simulink model "model_line_detector_2"  (R2023a)
settings: Solver=VariableStepAuto  StartTime=0.0  StopTime=25  RelTol=1e-3
model workspace (MAT data in the model file):
  BusActorsActors = canlib.Parameter
  BusActorsActors.DataType = 'auto'
  BusActorsActors.Complexity = 'real'
  BusActorsActors.Dimensions = [0 0]
values from neighbouring files (symbols this model uses):
  A = [a11 a12 ... (first row only)    [model.m]
  af = 1.104    [calc_Kvar.m]    (also in model.m)
  B = [b11 b12 ... (first row only)    [model.m]
  C = [1 0 ... (first row only)    [calc_Kvar.m]    (also in model.m)
  D = [0 0;0 0]    [calc_Kvar.m]    (also in model.m)
  E = [e1 ... (first row only)    [model.m]
  x0 = [0; 0]    [model.m]
undefined symbols (not defined in the file or in its folder): calc_A, calc_B, calc_E, calc_fb, calc_ff, driving, sigbuilder_block
libraries: drivingscenarioandsensors x2
settings Model: PacingRate=2  Creator=Utente  LastModifiedBy=Ferna
settings SolverCC: AlgebraicLoopSolver=TrustRegion
settings DebuggingCC: UnconnectedInputMsg=warning  UnconnectedOutputMsg=warning  UnconnectedLineMsg=warning
settings ModelReferenceCC: EnableRefExpFcnMdlSchedulingChecks=on
settings RTWCC: DLArmComputeVersion=19.05

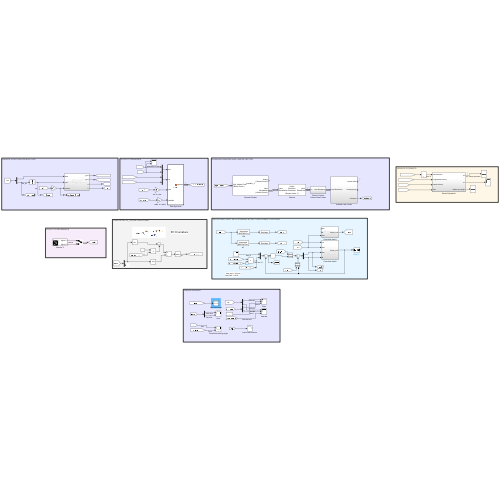
[thumbnail: Simulink's stored preview of the top-level diagram]
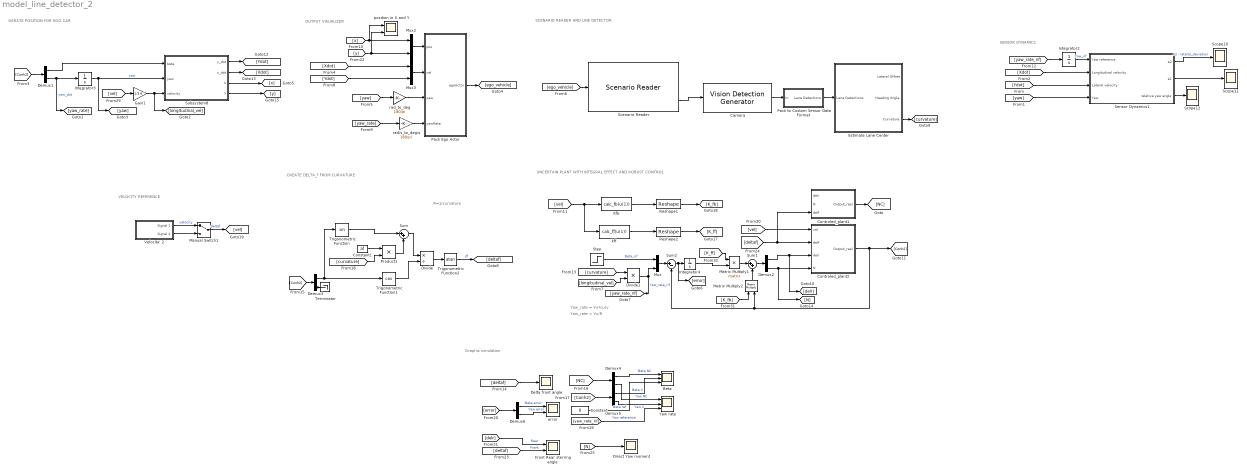
== system model_line_detector_2 ==
  note: Graphis simulation
  note: VELOCITY REFERENCE
  note: GERATE POSITION FOR EGO CAR
  note: UNCERTAIN PLANT WITH INTEGRAL EFFECT AND ROBUST CONTROL
  note: CREATE DELTA_f FROM CURVATURE
  note: SCENARIO READER AND LINE DETECTOR
  note: Yaw_rate = Vx*curv
  note: Yaw_rate = Vx/R
  note: SENSOR DYNAMICS
  note: OUTPUT VISUALIZER
  note: R=1/curvature
  Beta : Scope  NumInputPorts=3
  Camera : drivingscenarioandsensors/Vision Detection Generator  SensorIndex=1  DetectorOutput=Lanes only  UpdateInterval=0.01  LaneUpdateInterval=0.1  SensorLocation=[1.9 0]  Height=1.1  Yaw=0  Pitch=1  Roll=0  BusNameSource=Auto  BusName=BusObjectDetections  BusName2Source=Property  BusName2=BusVision  MaxNumDetectionsSource=Property  MaxNumDetections=50  MaxNumLanesSource=Property  MaxNumLanes=2  DetectionCoordinates=Ego Cartesian  SimulateUsing=Interpreted execution  MaxRange=50  BoundingBoxAccuracy=5  ProcessNoiseIntensity=5  MaxSpeed=50  MaxAllowedOcclusion=0.5  MinObjectImageSize=[15 15]  DetectionProbability=0.9  FalsePositivesPerImage=0.1  MinLaneImageSize=[20 3]  LaneBoundaryAccuracy=3  HasNoise=on  InitialSeedSource=Specify seed  InitialSeed=0  UsedSeed=0  ActorProfilesSource=Parameters  ActorProfilesParameters=driving.internal.ActorProfilesParameters  ActorProfilesExpression=[struct('ActorID',1,'ClassID',1,'Length',4.7,'Width',1.8,'Height',1.4,'OriginOffset',[-1.35 0 0],'MeshVertices',[3.7 -0.9 1.4;3.7 0.9 1.4;-1 0.9 1.4;-1 -0.9 1.4;3.7 -0.9 0;3.7 0.9 0;-1 0.9 0;-1 -0.9 0],'MeshFaces',[6 2 1;1 5 6;8 4 3;3 7 8;6 7 3;3 2 6;5 1 4;4 8 5;4 1 2;2 3 4;7 6 5;5 8 7],'RCSPattern',[10 10;10 10],'RCSAzimuthAngles',[-180 180],'RCSElevationAngles',[-90 90])]  Intrinsics=driving.internal.cameraIntrinsics('FocalLength',[800 799.999999999999],'PrincipalPoint',[320 240],'ImageSize',[480 640],'RadialDistortion',[0 0],'TangentialDistortion',[0 0],'Skew',0)
  Constant : Constant  Value=0
  Constant1 : Constant  Value=af
  Controled_plant1 : Subsystem
  Controled_plant2 : Subsystem
  Delta front angle : Scope
  Demux{1..6} (6 alike) : Demux  Outputs=2
  Direct Yaw moment : Scope
  Divide : Product  Inputs=*/
  Divide1 : Product  Inputs=**
  Estimate Lane Center : Subsystem  VariantControl=v2
  Front Rear sterring angle : Scope  NumInputPorts=2
  Gain1 : Gain  Gain=1/3.6
  Integrator2 : Integrator
  Integrator3 : Integrator  InitialCondition=0 %0.5411
  Integrator4 : Integrator
  Kfb : MATLABFcn  MATLABFcn=calc_fb(u(1))
  Manual Switch1 : ManualSwitch
  Matrix Multiply1 : Product  Multiplication=Matrix(*)
  Matrix Multiply2 : Product  Multiplication=Matrix(*)
  Mux : Mux  Inputs=2
  Mux2 : Mux  Inputs=2
  Mux3 : Mux  Inputs=2
  Pack Ego Actor : MATLAB Function  TreatAsAtomicUnit=on
  Pack to Custom Sensor Data Format : Subsystem
  Product1 : Product
  Reshape1 : Reshape  OutputDimensionality=Customize  OutputDimensions=[2,2]
  Reshape2 : Reshape  OutputDimensionality=Customize  OutputDimensions=[2,2]
  Scenario Reader : drivingscenarioandsensors/Scenario Reader  ScenarioSource=From file  ScenarioFileName=C:\Users\Ferna\Desktop\MASTER\third semester\vehicle control\proyectos\Vehicle control Mod_2 MIO\matlab\scenario_2.mat  ScenarioVariableName=scenario  OutputCoordinateSystem=Vehicle coordinates  EgoVehicleSource=Input port  EgoVehicleActorID=1  OrientVehiclesOnRoad=off  OutputEgoVehiclePose=off  OutputEgoVehicleState=off  SampleTime=0.1  LaneBoundaryOutput=Ego vehicle lane boundaries  LaneBoundaryDistance=linspace(-150, 150, 1500)  LaneBoundaryLocation=Center of lane markings  BusNameSource=Auto  BusName=BusActors  BusNumActorsSource=Scenario  BusNumActors=100  BusName2Source=Auto  BusName2=BusLaneBoundaries  BusNumLaneBoundariesSource=Scenario  BusNumLaneBoundaries=10  BusName3Source=Auto  BusName3=BusEgoActor  BusName4Source=Auto  BusName4=BusEgoState  ShowCoordinateLabels=on  SimulateUsing=Interpreted execution
  Scope10 : Scope
  Scope11 : Scope
  Scope12 : Scope
  Sensor Dynamics1 : Subsystem
  Step : Step  After=0  SampleTime=0
  Subsystem8 : Subsystem
  Sum : Sum  Inputs=|++
  Sum1 : Sum  Inputs=|++
  Sum2 : Sum  Inputs=|+-
  Terminator : Terminator
  Trigonometric Function : Trigonometry
  Trigonometric Function1 : Trigonometry  Operator=cos
  Trigonometric Function2 : Trigonometry  Operator=atan
  Velocita' 2 : Subsystem  Tag=STV Subsys  LoadFcn=sigbuilder_block('load');  StartFcn=sigbuilder_block('start');  StopFcn=sigbuilder_block('stop');  ClipboardFcn=sigbuilder_block('clipboard');  mask(Sigbuilder block){tuvar=[0:10]}
      mask help: Simulink:masks:SigbuilderBlock_MD
      mask init:
      | if ~strcmp(get_param(bdroot(gcbh),'SimulationStatus'),'stopped') tuvar = sigbuilder_block('maskInit'); end
      settings: CopyFcn=sigbuilder_block('copy');  DeleteFcn=sigbuilder_block('delete');  ModelCloseFcn=sigbuilder_block('modelClose');  PreSaveFcn=sigbuilder_block('preSave');  PauseFcn=sigbuilder_block('pause');  ContinueFcn=sigbuilder_block('continue');  NameChangeFcn=sigbuilder_block('namechange');  OpenFcn=sigbuilder_block('open',[5.4 36 1141.2 516.6 ]);  CloseFcn=sigbuilder_block('close');
      mask Display: plot(0, 0, 100, 100,[2, 2, 32, 32, 2], [68, 8, 8, 68, 68],[32, 2], [38, 38], [32, 19, 2],[53, 60, 44], [32, 17, 17, 2],[16, 16, 31, 31]);txt = getActiveGroup(gcbh);text(2, 100, txt,'verticalAlignment', 'top');
  Yaw rate : Scope  NumInputPorts=3
  error : Scope  NumInputPorts=2
  kff : MATLABFcn  MATLABFcn=calc_ff(u(1))
  position in X and Y : Scope  NumInputPorts=2
  rad/s_to_deg/s : Gain  Gain=180/pi
  "rad_to_deg  " : Gain  Gain=180/pi
  wires:
  [Xdot] -> Sensor Dynamics1/2(Longitudinal velocity)
  [Ydot] -> Sensor Dynamics1/3(Lateral velocity)
  [yaw] -> Sensor Dynamics1/4("Yaw ")
  Mux2/1 -> Pack Ego Actor/1(pos)
  [Xdot] -> Mux3/1
  Mux3/1 -> Pack Ego Actor/2(vel)
  [yaw] -> "rad_to_deg  "/1
  Pack Ego Actor/1(egoActor) -> [ego_vehicle]
  [yaw_rate] -> rad/s_to_deg/s/1
  "rad_to_deg  "/1 -> Pack Ego Actor/3(yaw)
  [Ydot] -> Mux3/2
  rad/s_to_deg/s/1 -> Pack Ego Actor/4(yawRate)
  [x] -> position in X and Y/1, Mux2/1
  [y] -> Mux2/2, position in X and Y/2
  Camera/1 -> Pack to Custom Sensor Data Format/1(In)
  Scenario Reader/2 -> Camera/1
  Pack to Custom Sensor Data Format/1(Lane Detections) -> Estimate Lane Center/1(Lane Detections)
  [ego_vehicle] -> Scenario Reader/1
  Divide1/1 -> [yaw_rate_rif], Mux/2  "Yaw_rate_rif"
  Estimate Lane Center/3(" Curvature") -> [curvature]
  Integrator2/1 -> Sensor Dynamics1/1(Yaw reference)  "Yaw_rif"
  [longitudinal_vel] -> Divide1/2
  Sensor Dynamics1/1(e2) -> Scope10/1  "e2 - lateral_deviation"
  Subsystem8/1(y_dot) -> [Ydot]
  Gain1/1 -> [longitudinal_vel], Subsystem8/3(velocity)
  Sensor Dynamics1/2(e1) -> Scope11/1
  Sensor Dynamics1/3(relative yaw angle) -> Scope12/1
  Demux2/2 -> [N], Controled_plant2/4(N)
  [deltaf] -> Controled_plant1/3(delf), Controled_plant2/2(delf)
  Matrix Multiply1/1 -> Sum1/1
  Demux2/1 -> [delr], Controled_plant2/3(delr)
  Sum2/1 -> [error], Integrator4/1
  Sum1/1 -> Demux2/1
  Controled_plant2/1(Output_real) -> Sum2/2, Matrix Multiply2/2, [Conh2]
  Controled_plant1/1(Output_real) -> [NC]
  Integrator4/1 -> Matrix Multiply1/2
  Demux3/2 -> Terminator/1
  Demux1/1 -> Subsystem8/1(beta)
  Demux1/2 -> [yaw_rate], Integrator3/1  "yaw_dot"
  Integrator3/1 -> [yaw], Subsystem8/2(yaw)  "yaw"
  Subsystem8/2(x_dot) -> [Xdot]
  Subsystem8/3(X) -> [x]
  Subsystem8/4(Y) -> [y]
  Mux/1 -> Sum2/1
  Step/1 -> Mux/1  "Beta_rif"
  [Conh2] -> Demux1/1
  [Conh2] -> Demux3/1
  Reshape2/1 -> [K_ff]
  [vel] -> Gain1/1
  [K_fb] -> Matrix Multiply2/1
  Matrix Multiply2/1 -> Sum1/2
  [vel] -> Controled_plant2/1(vel)
  Reshape1/1 -> [K_fb]
  [K_ff] -> Matrix Multiply1/1
  [vel] -> kff/1, Kfb/1
  Kfb/1 -> Reshape1/1
  kff/1 -> Reshape2/1
  Velocita' 2/1(Signal 1) -> Manual Switch1/1  "velocity"
  Velocita' 2/2(Signal 2) -> Manual Switch1/2
  Manual Switch1/1 -> [vel]  "deltaf"
  [curvature] -> Divide1/1
  Trigonometric Function1/1 -> Divide/2
  Product1/1 -> Sum/2
  Constant1/1 -> Product1/1
  Trigonometric Function/1 -> Sum/1
  [curvature] -> Product1/2
  Trigonometric Function2/1 -> [deltaf]  "df"
  Demux3/1 -> Trigonometric Function/1, Trigonometric Function1/1
  Sum/1 -> Divide/1
  Divide/1 -> Trigonometric Function2/1
  [yaw_rate_rif] -> Integrator2/1
  [deltaf] -> Delta front angle/1
  [NC] -> Demux4/1
  [Conh2] -> Demux5/1
  Demux4/1 -> Beta/1  "Beta NC"
  Demux5/1 -> Beta/2  "Beta C"
  Constant/1 -> Beta/3  "Beta ref"
  Demux4/2 -> Yaw rate/1  "Yaw NC"
  Demux5/2 -> Yaw rate/2  "Yaw C"
  [yaw_rate_rif] -> Yaw rate/3  "Yaw reference"
  [error] -> Demux6/1
  Demux6/1 -> error/1  "Beta error"
  Demux6/2 -> error/2  "Yaw error"
  [delr] -> Front Rear sterring angle/1  "Rear"
  [deltaf] -> Front Rear sterring angle/2  "Front"
  [N] -> Direct Yaw moment/1

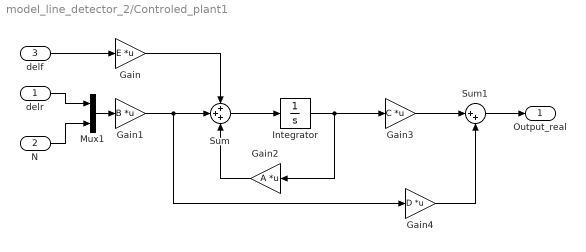
== system model_line_detector_2/Controled_plant1 ==
  delr : Inport
  N : Inport  Port=2
  delf : Inport  Port=3
  Gain : Gain  Gain=E  Multiplication=Matrix(K*u)
  Gain1 : Gain  Gain=B  Multiplication=Matrix(K*u)
  Gain2 : Gain  Gain=A  Multiplication=Matrix(K*u)
  Gain3 : Gain  Gain=C  Multiplication=Matrix(K*u)
  Gain4 : Gain  Gain=D  Multiplication=Matrix(K*u)
  Integrator : Integrator  InitialCondition=x0
  Mux1 : Mux  Inputs=2
  Sum : Sum  Inputs=+++
  Sum1 : Sum  Inputs=|++
  Output_real : Outport
  wires:
  Gain2/1 -> Sum/3
  Sum/1 -> Integrator/1
  Mux1/1 -> Gain1/1
  N/1 -> Mux1/2
  Gain3/1 -> Sum1/1
  Sum1/1 -> Output_real/1
  Gain/1 -> Sum/1
  Integrator/1 -> Gain2/1, Gain3/1
  delf/1 -> Gain/1
  delr/1 -> Mux1/1
  Gain4/1 -> Sum1/2
  Gain1/1 -> Sum/2, Gain4/1

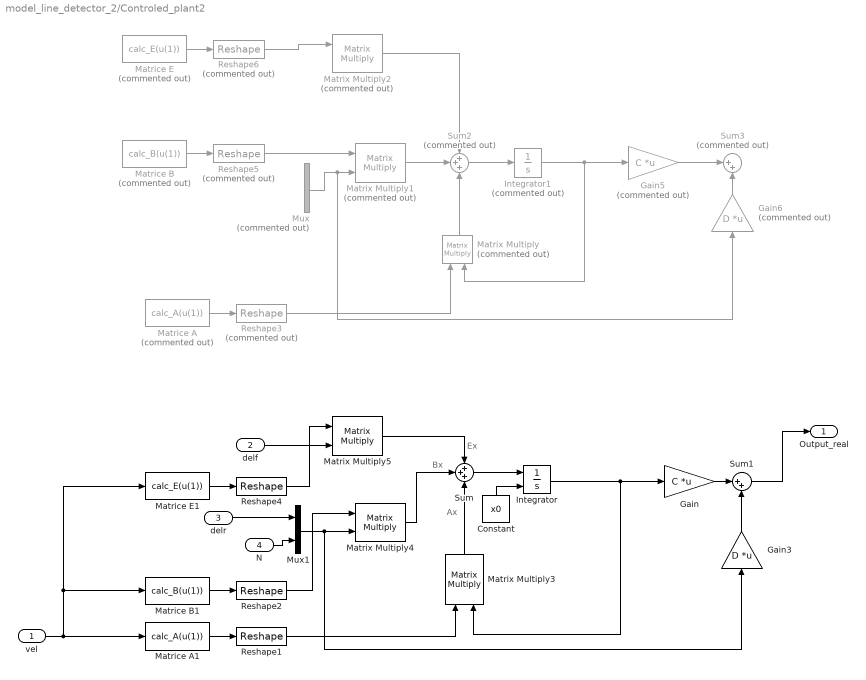
== system model_line_detector_2/Controled_plant2 ==
  note: Ex
  note: Bx
  note: Ax
  vel : Inport
  delf : Inport  Port=2
  delr : Inport  Port=3
  N : Inport  Port=4
  Constant : Constant  Value=x0
  Gain : Gain  Gain=C  Multiplication=Matrix(K*u)
  Gain3 : Gain  Gain=D  Multiplication=Matrix(K*u)
  Gain5 : Gain  Commented=on  Gain=C  Multiplication=Matrix(K*u)
  Gain6 : Gain  Commented=on  Gain=D  Multiplication=Matrix(K*u)
  Integrator : Integrator  InitialConditionSource=external
  Integrator1 : Integrator  Commented=on  InitialCondition=x0
  Matrice A : MATLABFcn  Commented=on  MATLABFcn=calc_A(u(1))
  Matrice A1 : MATLABFcn  MATLABFcn=calc_A(u(1))
  Matrice B : MATLABFcn  Commented=on  MATLABFcn=calc_B(u(1))
  Matrice B1 : MATLABFcn  MATLABFcn=calc_B(u(1))
  Matrice E : MATLABFcn  Commented=on  MATLABFcn=calc_E(u(1))
  Matrice E1 : MATLABFcn  MATLABFcn=calc_E(u(1))
  Matrix Multiply : Product  Commented=on  Multiplication=Matrix(*)
  Matrix Multiply1 : Product  Commented=on  Multiplication=Matrix(*)
  Matrix Multiply2 : Product  Commented=on  Multiplication=Matrix(*)
  Matrix Multiply3 : Product  Multiplication=Matrix(*)
  Matrix Multiply4 : Product  Multiplication=Matrix(*)
  Matrix Multiply5 : Product  Multiplication=Matrix(*)
  Mux : Mux  Commented=on  Inputs=2
  Mux1 : Mux  Inputs=2
  Reshape1 : Reshape  OutputDimensionality=Customize  OutputDimensions=[2,2]
  Reshape2 : Reshape  OutputDimensionality=Customize  OutputDimensions=[2,2]
  Reshape3 : Reshape  Commented=on  OutputDimensionality=Customize  OutputDimensions=[2,2]
  Reshape4 : Reshape  OutputDimensionality=Customize  OutputDimensions=[2,1]
  Reshape5 : Reshape  Commented=on  OutputDimensionality=Customize  OutputDimensions=[2,2]
  Reshape6 : Reshape  Commented=on  OutputDimensionality=Customize  OutputDimensions=[2,1]
  Sum : Sum  Inputs=+++
  Sum1 : Sum  Inputs=|++
  Sum2 : Sum  Commented=on  Inputs=+++
  Sum3 : Sum  Commented=on  Inputs=|++
  Output_real : Outport
  wires:
  Matrice E/1 -> Reshape6/1
  Reshape6/1 -> Matrix Multiply2/1
  Matrix Multiply1/1 -> Sum2/2
  Mux/1 -> Gain6/1, Matrix Multiply1/2
  Reshape3/1 -> Matrix Multiply/1
  Matrice A/1 -> Reshape3/1
  Gain5/1 -> Sum3/1
  Gain6/1 -> Sum3/2
  Integrator1/1 -> Gain5/1, Matrix Multiply/2
  Sum2/1 -> Integrator1/1
  Matrix Multiply2/1 -> Sum2/1
  Matrix Multiply/1 -> Sum2/3
  Matrice B/1 -> Reshape5/1
  Reshape5/1 -> Matrix Multiply1/1
  Matrix Multiply3/1 -> Sum/3
  delf/1 -> Matrix Multiply5/2
  Mux1/1 -> Gain3/1, Matrix Multiply4/2
  Gain3/1 -> Sum1/2
  Reshape2/1 -> Matrix Multiply4/1
  Matrix Multiply5/1 -> Sum/1
  Matrice A1/1 -> Reshape1/1
  Matrice E1/1 -> Reshape4/1
  Gain/1 -> Sum1/1
  vel/1 -> Matrice A1/1, Matrice E1/1, Matrice B1/1
  Sum/1 -> Integrator/1
  Reshape4/1 -> Matrix Multiply5/1
  Matrix Multiply4/1 -> Sum/2
  Integrator/1 -> Matrix Multiply3/2, Gain/1
  delr/1 -> Mux1/1
  Reshape1/1 -> Matrix Multiply3/1
  Matrice B1/1 -> Reshape2/1
  Constant/1 -> Integrator/2
  Sum1/1 -> Output_real/1
  N/1 -> Mux1/2

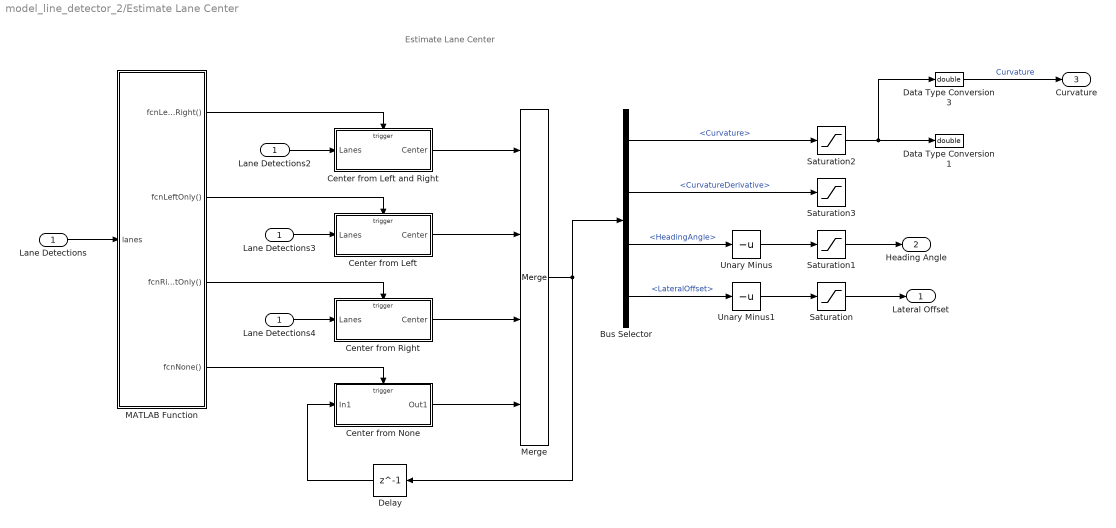
== system model_line_detector_2/Estimate Lane Center ==
  note: Estimate Lane Center
  Lane Detections : Inport
  Bus Selector : BusSelector  OutputSignals=Curvature,CurvatureDerivative,HeadingAngle,LateralOffset
  Center from Left : Subsystem  TreatAsAtomicUnit=on
  Center from Left and Right : Subsystem  TreatAsAtomicUnit=on
  Center from None : Subsystem  TreatAsAtomicUnit=on
  Center from Right : Subsystem  TreatAsAtomicUnit=on
  Data Type Conversion1 : DataTypeConversion  OutDataTypeStr=double  SaturateOnIntegerOverflow=off  RndMeth=Floor
  Data Type Conversion3 : DataTypeConversion  OutDataTypeStr=double  SaturateOnIntegerOverflow=off  RndMeth=Floor
  Delay : Delay  DelayLength=1
  Lane Detections2 : InportShadow
  Lane Detections3 : InportShadow
  Lane Detections4 : InportShadow
  MATLAB Function : MATLAB Function  TreatAsAtomicUnit=on
  Merge : Merge  Inputs=4
  Saturation : Saturate  UpperLimit=inf
  Saturation1 : Saturate  UpperLimit=0.6  LowerLimit=-0.6
  Saturation2 : Saturate  UpperLimit=0.15  LowerLimit=-0.15
  Saturation3 : Saturate  UpperLimit=0.15  LowerLimit=-0.15
  Unary Minus : UnaryMinus
  Unary Minus1 : UnaryMinus
  Lateral Offset : Outport  VectorParamsAs1DForOutWhenUnconnected=off
  Heading Angle : Outport  Port=2  VectorParamsAs1DForOutWhenUnconnected=off
  " Curvature" : Outport  Port=3  VectorParamsAs1DForOutWhenUnconnected=off
  wires:
  Center from Right/1(Center) -> Merge/3
  Lane Detections3/1 -> Center from Left/1(Lanes)
  Lane Detections4/1 -> Center from Right/1(Lanes)
  MATLAB Function/2(fcnLeftOnly()) -> Center from Left/Trigger
  Center from None/1(Out1) -> Merge/4
  MATLAB Function/1(fcnLeftAndRight()) -> Center from Left and Right/Trigger
  Delay/1 -> Center from None/1(In1)
  Center from Left and Right/1(Center) -> Merge/1
  Lane Detections/1 -> MATLAB Function/1(lanes)
  Lane Detections2/1 -> Center from Left and Right/1(Lanes)
  MATLAB Function/3(fcnRightOnly()) -> Center from Right/Trigger
  MATLAB Function/4(fcnNone()) -> Center from None/Trigger
  Center from Left/1(Center) -> Merge/2
  Merge/1 -> Bus Selector/1, Delay/1
  Saturation2/1 -> Data Type Conversion1/1, Data Type Conversion3/1
  Saturation1/1 -> Heading Angle/1
  Saturation/1 -> Lateral Offset/1
  Unary Minus/1 -> Saturation1/1
  Bus Selector/2 -> Saturation3/1  "<CurvatureDerivative>"
  Bus Selector/1 -> Saturation2/1  "<Curvature>"
  Unary Minus1/1 -> Saturation/1
  Bus Selector/4 -> Unary Minus1/1  "<LateralOffset>"
  Bus Selector/3 -> Unary Minus/1  "<HeadingAngle>"
  Data Type Conversion3/1 -> " Curvature"/1  "Curvature"

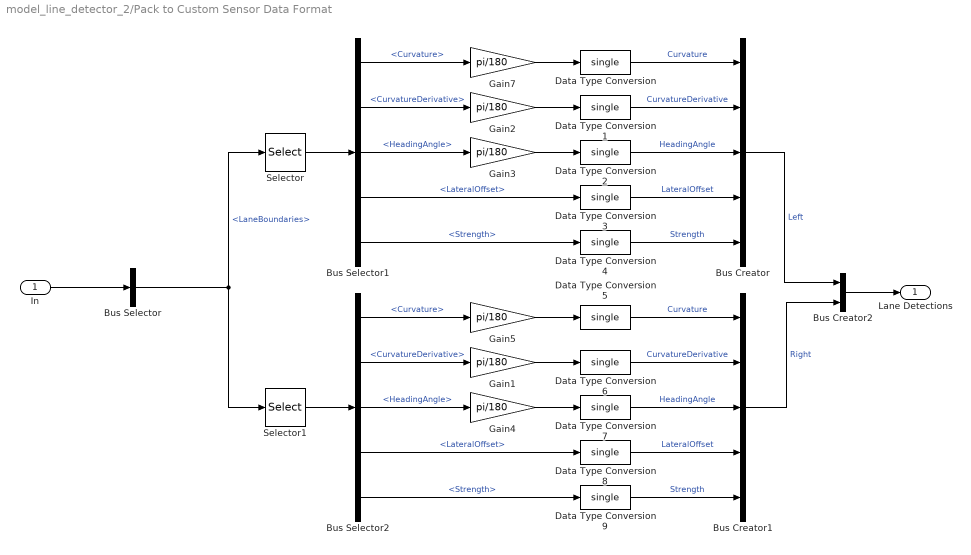
== system model_line_detector_2/Pack to Custom Sensor Data Format ==
  In : Inport
  Bus Creator : BusCreator  Inputs=5  OutDataTypeStr=Bus: LaneSensorBoundaries
  Bus Creator1 : BusCreator  Inputs=5  OutDataTypeStr=Bus: LaneSensorBoundaries
  Bus Creator2 : BusCreator  Inputs=2  OutDataTypeStr=Bus: LaneSensor
  Bus Selector : BusSelector  OutputSignals=LaneBoundaries
  Bus Selector1 : BusSelector  OutputSignals=Curvature,CurvatureDerivative,HeadingAngle,LateralOffset,Strength
  Bus Selector2 : BusSelector  OutputSignals=Curvature,CurvatureDerivative,HeadingAngle,LateralOffset,Strength
  Data Type Conversion{,1..9} (10 alike) : DataTypeConversion  OutDataTypeStr=single  SaturateOnIntegerOverflow=off  RndMeth=Floor
  Gain{1..5,7} (6 alike) : Gain  Gain=pi/180
  Selector : Selector  InputPortWidth=2  IndexOptions=Index vector (dialog)  Indices=1  OutputSizes=1
  Selector1 : Selector  InputPortWidth=2  IndexOptions=Index vector (dialog)  Indices=2  OutputSizes=1
  Lane Detections : Outport  VectorParamsAs1DForOutWhenUnconnected=off
  wires:
  In/1 -> Bus Selector/1
  Bus Selector/1 -> Selector/1, Selector1/1  "<LaneBoundaries>"
  Selector/1 -> Bus Selector1/1
  Bus Selector1/2 -> Gain2/1  "<CurvatureDerivative>"
  Bus Selector1/1 -> Gain7/1  "<Curvature>"
  Bus Selector1/3 -> Gain3/1  "<HeadingAngle>"
  Gain7/1 -> Data Type Conversion/1
  Gain2/1 -> Data Type Conversion1/1
  Gain3/1 -> Data Type Conversion2/1
  Bus Selector1/4 -> Data Type Conversion3/1  "<LateralOffset>"
  Bus Selector1/5 -> Data Type Conversion4/1  "<Strength>"
  Data Type Conversion/1 -> Bus Creator/1  "Curvature"
  Data Type Conversion1/1 -> Bus Creator/2  "CurvatureDerivative"
  Data Type Conversion2/1 -> Bus Creator/3  "HeadingAngle"
  Data Type Conversion3/1 -> Bus Creator/4  "LateralOffset"
  Data Type Conversion4/1 -> Bus Creator/5  "Strength"
  Data Type Conversion9/1 -> Bus Creator1/5  "Strength"
  Data Type Conversion6/1 -> Bus Creator1/2  "CurvatureDerivative"
  Data Type Conversion7/1 -> Bus Creator1/3  "HeadingAngle"
  Data Type Conversion8/1 -> Bus Creator1/4  "LateralOffset"
  Data Type Conversion5/1 -> Bus Creator1/1  "Curvature"
  Bus Selector2/1 -> Gain5/1  "<Curvature>"
  Selector1/1 -> Bus Selector2/1
  Bus Selector2/4 -> Data Type Conversion8/1  "<LateralOffset>"
  Bus Selector2/5 -> Data Type Conversion9/1  "<Strength>"
  Bus Selector2/2 -> Gain1/1  "<CurvatureDerivative>"
  Gain4/1 -> Data Type Conversion7/1
  Gain5/1 -> Data Type Conversion5/1
  Gain1/1 -> Data Type Conversion6/1
  Bus Selector2/3 -> Gain4/1  "<HeadingAngle>"
  Bus Creator2/1 -> Lane Detections/1
  Bus Creator/1 -> Bus Creator2/1  "Left"
  Bus Creator1/1 -> Bus Creator2/2  "Right"

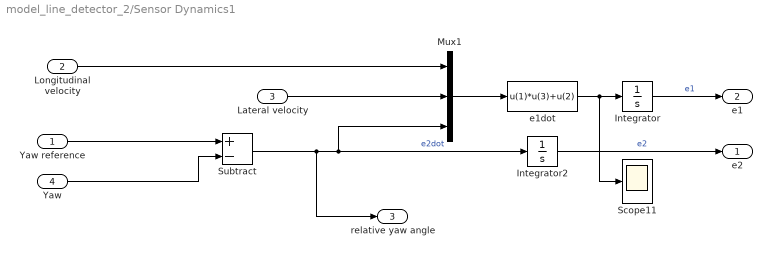
== system model_line_detector_2/Sensor Dynamics1 ==
  Yaw reference : Inport
  Longitudinal velocity : Inport  Port=2
  Lateral velocity : Inport  Port=3
  "Yaw " : Inport  Port=4
  Integrator : Integrator
  Integrator2 : Integrator
  Mux1 : Mux  Inputs=[1 1 1]
  Scope11 : Scope
  Subtract : Sum  Inputs=+-
  e1dot : Fcn  Expr=u(1)*u(3)+u(2)
  e2 : Outport  VectorParamsAs1DForOutWhenUnconnected=off
  e1 : Outport  Port=2  VectorParamsAs1DForOutWhenUnconnected=off
  relative yaw angle : Outport  Port=3  VectorParamsAs1DForOutWhenUnconnected=off
  wires:
  Integrator2/1 -> e2/1  "e2"
  Mux1/1 -> e1dot/1
  e1dot/1 -> Scope11/1, Integrator/1
  Longitudinal velocity/1 -> Mux1/1
  Lateral velocity/1 -> Mux1/2
  Yaw reference/1 -> Subtract/1
  "Yaw "/1 -> Subtract/2
  Subtract/1 -> relative yaw angle/1, Mux1/3, Integrator2/1  "e2dot"
  Integrator/1 -> e1/1  "e1"

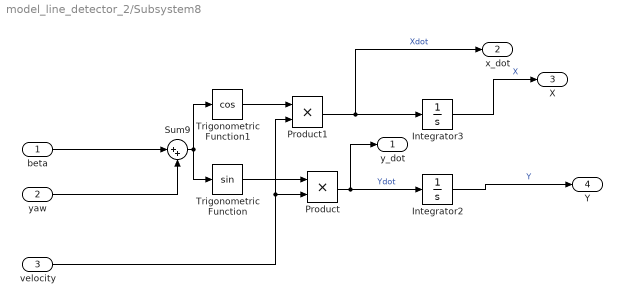
== system model_line_detector_2/Subsystem8 ==
  beta : Inport
  yaw : Inport  Port=2
  velocity : Inport  Port=3
  Integrator2 : Integrator  InitialCondition=0 %-130.88
  Integrator3 : Integrator  InitialCondition=0 %-284.47
  Product : Product
  Product1 : Product
  Sum9 : Sum  Inputs=|++
  Trigonometric Function : Trigonometry
  Trigonometric Function1 : Trigonometry  Operator=cos
  y_dot : Outport
  x_dot : Outport  Port=2
  X : Outport  Port=3
  Y : Outport  Port=4
  wires:
  Integrator3/1 -> X/1  "X"
  Product1/1 -> x_dot/1, Integrator3/1  "Xdot"
  velocity/1 -> Product1/2, Product/2
  yaw/1 -> Sum9/2
  Sum9/1 -> Trigonometric Function/1, Trigonometric Function1/1
  Trigonometric Function/1 -> Product/1
  Trigonometric Function1/1 -> Product1/1
  beta/1 -> Sum9/1
  Product/1 -> y_dot/1, Integrator2/1  "Ydot"
  Integrator2/1 -> Y/1  "Y"

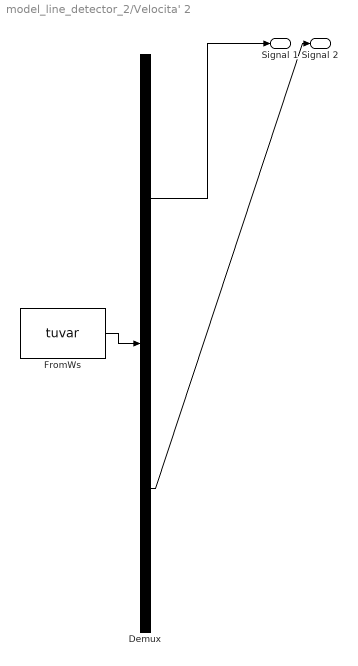
== system model_line_detector_2/Velocita' 2 ==
  Demux : Demux  Tag=STV Demux  Outputs=2
      settings: DisplayOption=none
  FromWs : FromWorkspace  Tag=STV FromWs  VariableName=tuvar
      SigBuilderData=|
      | common.afterFinalStr = 'Extrapolate'
      | common.sampleTime = 0
      | dataSet.timeRange = [0 45]
      | dataSet.name = 'Group 1'
      | sbobj.Groups.Name = 'Group 1'
      | sbobj.Groups.Signals(1).Name = 'Signal 1'
      | sbobj.Groups.Signals(1).XData = [0 4 6 10 12 16 18 22 24 30 34 45]
      | sbobj.Groups.Signals(1).YData = [51 51 58 58 66 66 66 81 81.2 81.2 70.2 70.2]
      | sbobj.Groups.Signals(2).Name = 'Signal 2'
      | sbobj.Groups.Signals(2).XData = [0 2.5 5 7.5 10 12.5 15 17.5 20 22.5 25 27.5 30 32.5 35 37.5 40 42.5 45]
      | sbobj.Groups.Signals(2).YData = [56 56 63 63 72 72 72 72 82 82 82 65 65 65 65 75.4 75.4 75.4 75.4]
      | sbobj.Groups.TimeRange = [0 45]
  Signal 1 : Outport  Tag=STV Outport
  Signal 2 : Outport  Tag=STV Outport  Port=2
  wires:
  FromWs/1 -> Demux/1
  Demux/1 -> Signal 1/1
  Demux/2 -> Signal 2/1

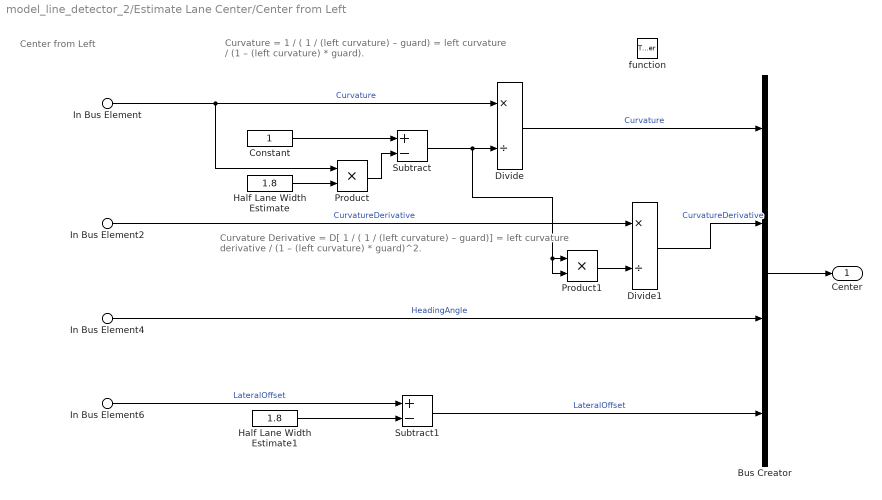
== system model_line_detector_2/Estimate Lane Center/Center from Left ==
  note: Curvature Derivative
      | = D[ 1 / ( 1 / (left curvature) – guard)]
      | = left curvature derivative / (1 – (left curvature) * guard)^2.
  note: Center from Left
  note: Curvature
      | = 1 / ( 1 / (left curvature) – guard)
      | = left curvature / (1 – (left curvature) * guard).
  In Bus Element : Inport  PortName=Lanes  Element=Left.Curvature
  In Bus Element2 : Inport  PortName=Lanes  Element=Left.CurvatureDerivative
  In Bus Element4 : Inport  PortName=Lanes  Element=Left.HeadingAngle
  In Bus Element6 : Inport  PortName=Lanes  Element=Left.LateralOffset
  function : TriggerPort  TriggerType=function-call  VariantControl=Variant
  Bus Creator : BusCreator  Inputs=4
  Constant : Constant  OutDataTypeStr=Inherit: Inherit via back propagation
  Divide : Product  Inputs=*/
  Divide1 : Product  Inputs=*/
  Half Lane Width Estimate : Constant  Value=1.8  OutDataTypeStr=Inherit: Inherit via back propagation
  Half Lane Width Estimate1 : Constant  Value=1.8  OutDataTypeStr=Inherit: Inherit via back propagation
  Product : Product
  Product1 : Product
  Subtract : Sum  Inputs=+-
  Subtract1 : Sum  Inputs=+-
  Center : Outport  VectorParamsAs1DForOutWhenUnconnected=off
  wires:
  Product/1 -> Subtract/2
  Half Lane Width Estimate1/1 -> Subtract1/2
  In Bus Element6/1 -> Subtract1/1  "LateralOffset"
  Product1/1 -> Divide1/2
  In Bus Element2/1 -> Divide1/1  "CurvatureDerivative"
  Constant/1 -> Subtract/1
  Half Lane Width Estimate/1 -> Product/2
  Subtract/1 -> Divide/2, Product1/1, Product1/2
  In Bus Element/1 -> Divide/1, Product/1  "Curvature"
  Subtract1/1 -> Bus Creator/4  "LateralOffset"
  In Bus Element4/1 -> Bus Creator/3  "HeadingAngle"
  Divide/1 -> Bus Creator/1  "Curvature"
  Divide1/1 -> Bus Creator/2  "CurvatureDerivative"
  Bus Creator/1 -> Center/1

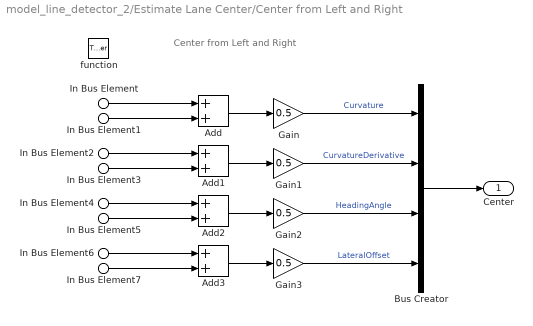
== system model_line_detector_2/Estimate Lane Center/Center from Left and Right ==
  note: Center from Left and Right
  In Bus Element : Inport  PortName=Lanes  Element=Left.Curvature
  In Bus Element2 : Inport  PortName=Lanes  Element=Left.CurvatureDerivative
  In Bus Element4 : Inport  PortName=Lanes  Element=Left.HeadingAngle
  In Bus Element6 : Inport  PortName=Lanes  Element=Left.LateralOffset
  In Bus Element1 : Inport  PortName=Lanes  Element=Right.Curvature
  In Bus Element3 : Inport  PortName=Lanes  Element=Right.CurvatureDerivative
  In Bus Element5 : Inport  PortName=Lanes  Element=Right.HeadingAngle
  In Bus Element7 : Inport  PortName=Lanes  Element=Right.LateralOffset
  function : TriggerPort  TriggerType=function-call  VariantControl=Variant
  Add{,1..3} (4 alike) : Sum
  Bus Creator : BusCreator  Inputs=4
  Gain{,1..3} (4 alike) : Gain  Gain=0.5
  Center : Outport  VectorParamsAs1DForOutWhenUnconnected=off
  wires:
  In Bus Element6/1 -> Add3/1
  In Bus Element7/1 -> Add3/2
  In Bus Element5/1 -> Add2/2
  In Bus Element4/1 -> Add2/1
  In Bus Element3/1 -> Add1/2
  In Bus Element2/1 -> Add1/1
  In Bus Element1/1 -> Add/2
  In Bus Element/1 -> Add/1
  Bus Creator/1 -> Center/1
  Gain3/1 -> Bus Creator/4  "LateralOffset"
  Add3/1 -> Gain3/1
  Gain2/1 -> Bus Creator/3  "HeadingAngle"
  Add2/1 -> Gain2/1
  Gain1/1 -> Bus Creator/2  "CurvatureDerivative"
  Add1/1 -> Gain1/1
  Gain/1 -> Bus Creator/1  "Curvature"
  Add/1 -> Gain/1

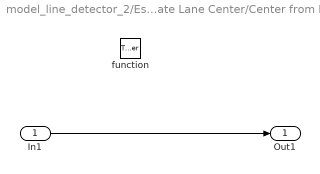
== system model_line_detector_2/Estimate Lane Center/Center from None ==
  In1 : Inport
  function : TriggerPort  TriggerType=function-call  VariantControl=Variant
  Out1 : Outport  VectorParamsAs1DForOutWhenUnconnected=off
  wires:
  In1/1 -> Out1/1

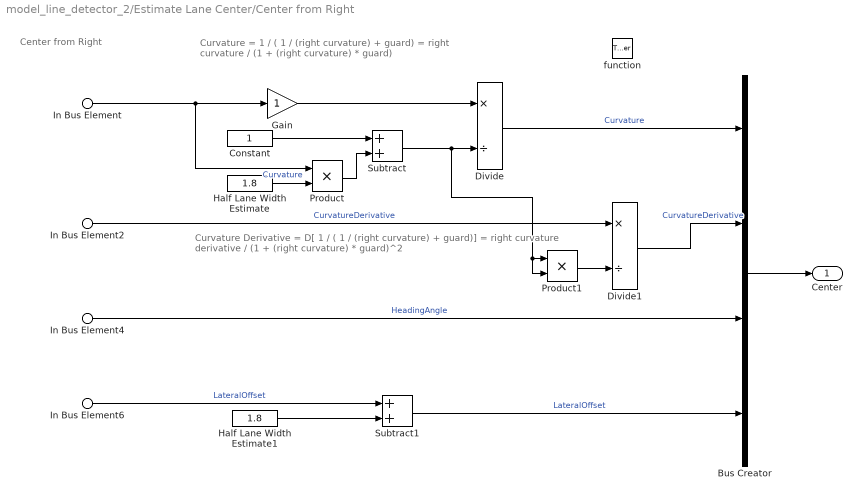
== system model_line_detector_2/Estimate Lane Center/Center from Right ==
  note: Curvature Derivative
      | = D[ 1 / ( 1 / (right curvature) + guard)]
      | = right curvature derivative / (1 + (right curvature) * guard)^2
  note: Curvature
      | = 1 / ( 1 / (right curvature) + guard)
      | = right curvature / (1 + (right curvature) * guard)
  note: Center from Right
  In Bus Element : Inport  PortName=Lanes  Element=Right.Curvature
  In Bus Element2 : Inport  PortName=Lanes  Element=Right.CurvatureDerivative
  In Bus Element4 : Inport  PortName=Lanes  Element=Right.HeadingAngle
  In Bus Element6 : Inport  PortName=Lanes  Element=Right.LateralOffset
  function : TriggerPort  TriggerType=function-call  VariantControl=Variant
  Bus Creator : BusCreator  Inputs=4
  Constant : Constant  OutDataTypeStr=Inherit: Inherit via back propagation
  Divide : Product  Inputs=*/
  Divide1 : Product  Inputs=*/
  Gain : Gain
  Half Lane Width Estimate : Constant  Value=1.8  OutDataTypeStr=Inherit: Inherit via back propagation
  Half Lane Width Estimate1 : Constant  Value=1.8  OutDataTypeStr=Inherit: Inherit via back propagation
  Product : Product
  Product1 : Product
  Subtract : Sum
  Subtract1 : Sum
  Center : Outport  VectorParamsAs1DForOutWhenUnconnected=off
  wires:
  Half Lane Width Estimate/1 -> Product/2
  Product/1 -> Subtract/2
  Constant/1 -> Subtract/1
  Subtract/1 -> Divide/2, Product1/1, Product1/2
  In Bus Element/1 -> Gain/1, Product/1  "Curvature"
  Bus Creator/1 -> Center/1
  Subtract1/1 -> Bus Creator/4  "LateralOffset"
  Divide/1 -> Bus Creator/1  "Curvature"
  In Bus Element6/1 -> Subtract1/1  "LateralOffset"
  Half Lane Width Estimate1/1 -> Subtract1/2
  In Bus Element4/1 -> Bus Creator/3  "HeadingAngle"
  Product1/1 -> Divide1/2
  Divide1/1 -> Bus Creator/2  "CurvatureDerivative"
  In Bus Element2/1 -> Divide1/1  "CurvatureDerivative"
  Gain/1 -> Divide/1

== matlab function model_line_detector_2/Pack Ego Actor ==
  data: pos input; egoActor output Bus: BusActors1Actors size=1; vel input; yaw input; yawRate input
function egoActor = packEgo(pos,vel,yaw,yawRate)
% Pack ego information into a single ego actor bus
%
% Imoprtant note:
% Output is a bus of type BusActorsActors. This is the same bus used by the
% Scenario Reader to output an individual actor. If you change the
% output bus name of Scenario Reader, change the output bus name here
% as well by clicking on 'Edit Data' in the menu above.

%Position x,y,z
%Velocity x,y,z
%Angular velocity wx, wy, wz

egoActor = struct(...
    'ActorID',1,...
    'Position', [pos(1) pos(2) 0], ...
    'Velocity', [vel(1) vel(2) 0], ...
    'Roll', 0, ...
    'Pitch', 0, ...
    'Yaw', yaw, ...
    'AngularVelocity', [0 0 yawRate]);

== matlab function model_line_detector_2/Estimate Lane Center/MATLAB Function ==
  data: lanes input
  events: fcnLeftAndRight output FUNCTION_CALL_EVENT; fcnLeftOnly output FUNCTION_CALL_EVENT; fcnRightOnly output FUNCTION_CALL_EVENT; fcnNone output FUNCTION_CALL_EVENT
function fcn(lanes)

leftStrength  = lanes.Left.Strength;
rightStrength = lanes.Right.Strength;

if (leftStrength > 0) && (rightStrength > 0)
   fcnLeftAndRight();
   
elseif leftStrength > 0
    fcnLeftOnly();
    
elseif rightStrength > 0
    fcnRightOnly();
    
else
    fcnNone();
end
